simulink library "GaitGenerationLibrary"  (R2016b)
settings: Solver=VariableStepAuto  StartTime=0.0  StopTime=10.0  RelTol=1e-3
settings Model: Creator=march  LastModifiedBy=march

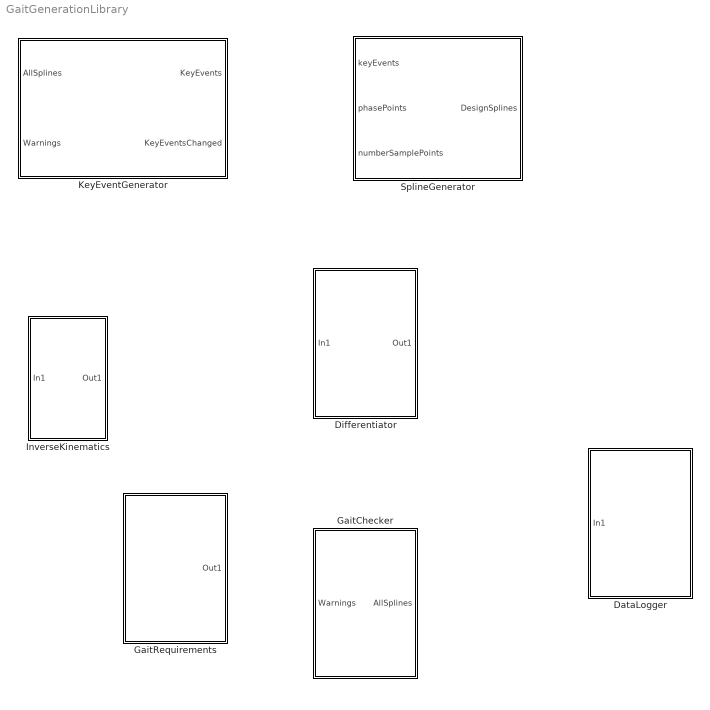
== system GaitGenerationLibrary ==
  DataLogger : Subsystem
  Differentiator : Subsystem
  GaitChecker : Subsystem
  GaitRequirements : Subsystem
  InverseKinematics : Subsystem
  KeyEventGenerator : Subsystem
  SplineGenerator : Subsystem

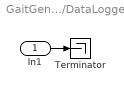
== system GaitGenerationLibrary/DataLogger ==
  In1 : Inport
  Terminator : Terminator
  wires:
  In1/1 -> Terminator/1

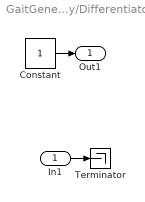
== system GaitGenerationLibrary/Differentiator ==
  In1 : Inport
  Constant : Constant
  Terminator : Terminator
  Out1 : Outport
  wires:
  Constant/1 -> Out1/1
  In1/1 -> Terminator/1

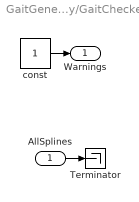
== system GaitGenerationLibrary/GaitChecker ==
  AllSplines : Inport
  Terminator : Terminator
  const : Constant
  Warnings : Outport
  wires:
  const/1 -> Warnings/1
  AllSplines/1 -> Terminator/1

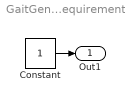
== system GaitGenerationLibrary/GaitRequirements ==
  Constant : Constant
  Out1 : Outport
  wires:
  Constant/1 -> Out1/1

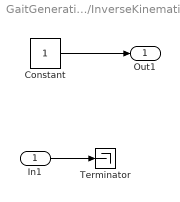
== system GaitGenerationLibrary/InverseKinematics ==
  In1 : Inport
  Constant : Constant
  Terminator : Terminator
  Out1 : Outport
  wires:
  In1/1 -> Terminator/1
  Constant/1 -> Out1/1

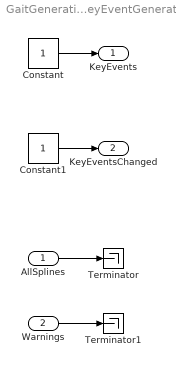
== system GaitGenerationLibrary/KeyEventGenerator ==
  AllSplines : Inport
  Warnings : Inport  Port=2
  Constant : Constant
  Constant1 : Constant
  Terminator : Terminator
  Terminator1 : Terminator
  KeyEvents : Outport
  KeyEventsChanged : Outport  Port=2
  wires:
  Constant/1 -> KeyEvents/1
  Constant1/1 -> KeyEventsChanged/1
  AllSplines/1 -> Terminator/1
  Warnings/1 -> Terminator1/1

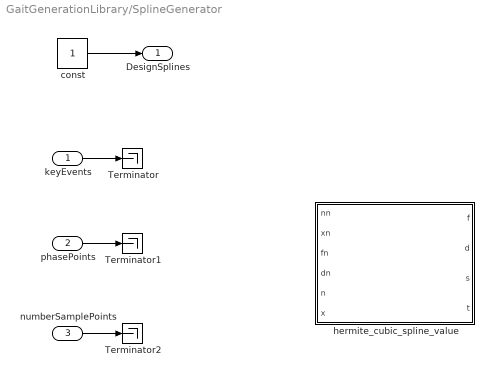
== system GaitGenerationLibrary/SplineGenerator ==
  keyEvents : Inport
  phasePoints : Inport  Port=2
  numberSamplePoints : Inport  Port=3
  Terminator : Terminator
  Terminator1 : Terminator
  Terminator2 : Terminator
  const : Constant
  hermite_cubic_spline_value : MATLAB Function  TreatAsAtomicUnit=on
  DesignSplines : Outport
  wires:
  keyEvents/1 -> Terminator/1
  const/1 -> DesignSplines/1
  phasePoints/1 -> Terminator1/1
  numberSamplePoints/1 -> Terminator2/1

== matlab function GaitGenerationLibrary/SplineGenerator/hermite_cubic_spline_value ==
  data: f output; d output; s output; nn input; xn input; fn input; dn input; n input; x input; t output
function [ f, d, s, t ] = hermite_cubic_spline_value( nn, xn, fn, dn, n, x )

%*****************************************************************************80
%
%% HERMITE_CUBIC_SPLINE_VALUE evaluates a Hermite cubic spline.
%
%  Licensing:
%
%    This code is distributed under the GNU LGPL license.
%
%  Modified:
%
%    27 January 2011
%
%  Author:
%
%    John Burkardt.
%
%  Reference:
%
%    Fred Fritsch, Ralph Carlson,
%    Monotone Piecewise Cubic Interpolation,
%    SIAM Journal on Numerical Analysis,
%    Volume 17, Number 2, April 1980, pages 238-246.
%
%  Parameters:
%
%    Input, integer NN, the number of data points.
%
%    Input, real XN(NN), the coordinates of the data points.
%    The entries in XN must be in strictly ascending order.
%
%    Input, real FN(NN), the function values.
%
%    Input, real DN(NN), the derivative values.
%
%    Input, integer N, the number of sample points.
%
%    Input, real X(N), the coordinates of the sample points.
%
%    Output, real F(N), the function value at the sample points.
%
%    Output, real D(N), the derivative value at the sample points.
%
%    Output, real S(N), the second derivative value at the sample points.
%
%    Output, real T(N), the third derivative value at the sample points.
%

%
%  Force data to be column vectors.
%
  xn = xn ( : );
  fn = fn ( : );
  dn = dn ( : );

  x = x ( : );
%
%  Insert "guard" values of -Inf and +Inf.
%
  xn2 = [ -Inf; xn(1:nn); +Inf ];
%
%  HISTC returns in I1 the index in XN2 such that
%  XN2(I1(I)) <= X(I) <= XN2(I1(I)+1).
%
  [ n1, i1 ] = histc ( x, xn2 );
%
%  Assign anything in the (-Inf,XN(1)) bin to (XN(1),XN(2)).
%
  k = find ( i1 == 1 );
  i1(k) = 2;
%
%  Assign anything in the (XN(NN),+Inf) bin to (XN(NN-1),XN(NN)).
%
  k = find ( i1 == nn + 1 );
  i1(k) = nn;
%
%  Now shift the indices down by 1 because -Inf is fictitious.
%
  i1 = i1 - 1;
%
%  Index the right hand endpoint.
%
  i2 = i1 + 1;
%
%  Evaluate the polynomial with the appropriate data.
%
  [ f, d, s, t ] = hermite_cubic_value ( xn(i1), fn(i1), dn(i1), ...
                                         xn(i2), fn(i2), dn(i2), n, x );

  return
end
